simulink model "MR11Simulinknodos"  (R2013a)
settings: Solver=ode45  StartTime=0.0  StopTime=10.0  RelTol=1e-3
libraries: powerlib x63
settings Model: Creator=Erika  LastModifiedBy=Erika

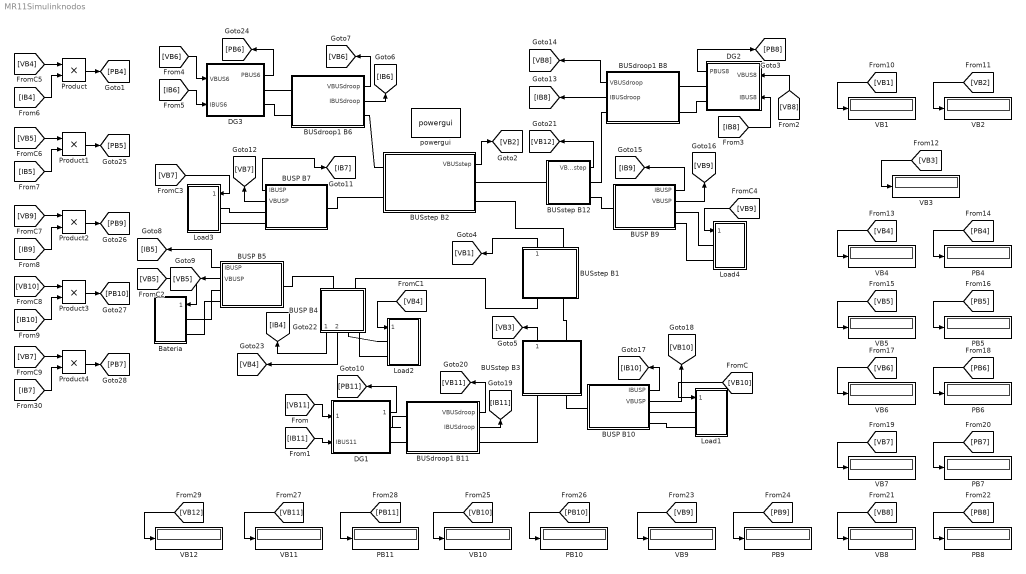
== system MR11Simulinknodos ==
  BUSP B10 : Subsystem
  BUSP B4 : Subsystem
  BUSP B5 : Subsystem
  BUSP B7 : Subsystem
  BUSP B9 : Subsystem
  BUSdroop1 B11 : Subsystem
  BUSdroop1 B6 : Subsystem
  BUSdroop1 B8 : Subsystem
  BUSstep B1 : Subsystem
  BUSstep B12 : Subsystem
  BUSstep B2 : Subsystem
  BUSstep B3 : Subsystem
  Bateria : Subsystem
  DG1 : Subsystem
  DG2 : Subsystem
  DG3 : Subsystem
  Load1 : Subsystem
  Load2 : Subsystem
  Load3 : Subsystem
  Load4 : Subsystem
  PB{4..11} (8 alike) : Display
  Product{,1..4} (5 alike) : Product
  VB{1..12} (12 alike) : Display
  powergui : powerlib/powergui  Priority=1  SimulationMode=Continuous  SolverType=Tustin  SampleTime=50e-6  frequency=60  SPID=off  DisableSnubberDevices=off  DisableRonSwitches=off  DisableVfSwitches=off  SwTol=0  Interpol=off  DisplayEquations=off  frequencyindice=0  Pbase=100e6  ErrMax=1e-4  Iterations=50  UnitsV=kV  UnitsW=MW  FunctionMessages=off  echomessages=off  HookPort=off  EnableUseOfTLC=off  x0status=blocks  RestoreLinks=warning  ResistiveCurrentMeasurement=off  Frange=[0:2:500]  Ylog=off  Xlog=on  ShowGrid=off  save=off  variable=ZData  ZoomFFT=off  StartTime=0.0  cycles=1  DisplayStyle=1  fundamental=60  FreqAxis=off  MaxFrequency=1000  frequencyindicesteady=1  RmsSteady=1  display=off  Ts=0  methode=off
  wires:
  [VB11] -> DG1/1(VBUS11)
  [IB11] -> DG1/2(IBUS11)
  DG1/1(PBUS11) -> [PB11]
  BUSP B5/1(IBUSP) -> [IB5]
  BUSP B5/2(VBUSP) -> [VB5]
  [VB10] -> Load1/1(VBUSc)
  BUSstep B1/1(VBUSstep) -> [VB1]
  BUSstep B2/1(VBUSstep) -> [VB2]
  BUSstep B3/1(VBUSstep) -> [VB3]
  BUSdroop1 B6/1(VBUSdroop) -> [VB6]
  BUSdroop1 B6/2(IBUSdroop) -> [IB6]
  BUSP B7/1(IBUSP) -> [IB7]
  BUSP B7/2(VBUSP) -> [VB7]
  BUSdroop1 B8/1(VBUSdroop) -> [VB8]
  BUSdroop1 B8/2(IBUSdroop) -> [IB8]
  BUSP B9/1(IBUSP) -> [IB9]
  BUSP B9/2(VBUSP) -> [VB9]
  BUSP B10/1(IBUSP) -> [IB10]
  BUSP B10/2(VBUSP) -> [VB10]
  BUSdroop1 B11/1(VBUSdroop) -> [VB11]
  BUSdroop1 B11/2(IBUSdroop) -> [IB11]
  BUSstep B12/1(VBUSstep) -> [VB12]
  BUSP B4/1(IBUSP) -> [IB4]
  BUSP B4/2(VBUSP) -> [VB4]
  [VB8] -> DG2/1(VBUS8)
  [IB8] -> DG2/2(IBUS8)
  DG2/1(PBUS8) -> [PB8]
  [VB6] -> DG3/1(VBUS6)
  [IB6] -> DG3/2(IBUS6)
  DG3/1(PBUS6) -> [PB6]
  [VB4] -> Load2/1(VBUSc)
  [VB5] -> Bateria/1(VBUSc)
  [VB7] -> Load3/1(VBUSc)
  [VB9] -> Load4/1(VBUSc)
  [VB4] -> Product/1
  [IB4] -> Product/2
  Product/1 -> [PB4]
  [VB5] -> Product1/1
  [IB5] -> Product1/2
  Product1/1 -> [PB5]
  [VB9] -> Product2/1
  [IB9] -> Product2/2
  Product2/1 -> [PB9]
  [VB10] -> Product3/1
  [IB10] -> Product3/2
  Product3/1 -> [PB10]
  [VB1] -> VB1/1
  [VB2] -> VB2/1
  [VB3] -> VB3/1
  [VB4] -> VB4/1
  [PB4] -> PB4/1
  [VB5] -> VB5/1
  [PB5] -> PB5/1
  [VB6] -> VB6/1
  [PB6] -> PB6/1
  [VB7] -> VB7/1
  [PB7] -> PB7/1
  [VB8] -> VB8/1
  [PB8] -> PB8/1
  [VB9] -> VB9/1
  [PB9] -> PB9/1
  [VB10] -> VB10/1
  [PB10] -> PB10/1
  [VB11] -> VB11/1
  [PB11] -> PB11/1
  [VB12] -> VB12/1
  [VB7] -> Product4/1
  [IB7] -> Product4/2
  Product4/1 -> [PB7]
  connections:
  BUSstep B1/RConn1 -- BUSstep B2/RConn2
  BUSstep B1/LConn1 -- BUSP B4/LConn2
  BUSstep B1/LConn2 -- BUSstep B3/RConn1
  BUSstep B2/RConn1 -- BUSstep B12/LConn1
  BUSstep B12/RConn2 -- BUSP B9/LConn1
  BUSstep B12/RConn1 -- BUSdroop1 B8/RConn1
  BUSstep B2/LConn1 -- BUSdroop1 B6/RConn1
  BUSstep B2/LConn2 -- BUSP B7/LConn1
  BUSP B4/LConn1 -- BUSP B5/LConn1
  BUSstep B3/LConn1 -- BUSdroop1 B11/RConn1
  BUSstep B3/LConn2 -- BUSP B10/LConn1
  DG1/RConn1 -- BUSdroop1 B11/LConn1
  DG1/RConn2 -- BUSdroop1 B11/LConn2
  DG2/RConn1 -- BUSdroop1 B8/LConn1
  DG2/RConn2 -- BUSdroop1 B8/LConn2
  DG3/RConn1 -- BUSdroop1 B6/LConn1
  DG3/RConn2 -- BUSdroop1 B6/LConn2
  Load1/LConn1 -- BUSP B10/RConn1
  Load1/LConn2 -- BUSP B10/RConn2
  Load2/LConn2 -- BUSP B4/RConn2
  Load2/LConn1 -- BUSP B4/RConn1
  Bateria/LConn1 -- BUSP B5/RConn1
  Bateria/LConn2 -- BUSP B5/RConn2
  Load3/LConn2 -- BUSP B7/RConn2
  Load3/LConn1 -- BUSP B7/RConn1
  Load4/LConn1 -- BUSP B9/RConn1
  Load4/LConn2 -- BUSP B9/RConn2

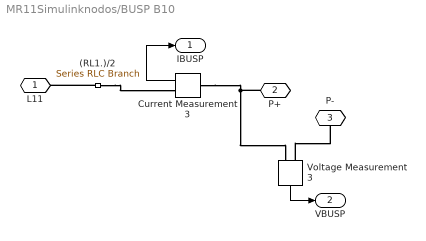
== system MR11Simulinknodos/BUSP B10 ==
  (RL1.)/2 : powerlib/Elements/Series RLC Branch  LConnTagsString=__new0  RConnTagsString=__new0  BranchType=R  Resistance=0.09  Inductance=1e-3  SetiL0=off  InitialCurrent=0  Capacitance=1e-6  Setx0=off  InitialVoltage=0  Measurements=None
  Current Measurement3 : powerlib/Measurements/Current Measurement  PhasorSimulation=off  OutputType=Complex  PSBequivalent=0
  Voltage Measurement3 : powerlib/Measurements/Voltage Measurement  PhasorSimulation=off  OutputType=Complex  PSBequivalent=0
  L11 : PMIOPort  Port=1  Side=Left
  P+ : PMIOPort  Port=2  Side=Right
  P- : PMIOPort  Port=3  Side=Right
  IBUSP : Outport
  VBUSP : Outport  Port=2
  wires:
  Current Measurement3/1 -> IBUSP/1
  Voltage Measurement3/1 -> VBUSP/1
  connections:
  Voltage Measurement3/LConn2 -- P-/RConn1
  (RL1.)/2/LConn1 -- L11/RConn1
  (RL1.)/2/RConn1 -- Current Measurement3/RConn1
  Current Measurement3/LConn1 -- Voltage Measurement3/LConn1 -- P+/RConn1

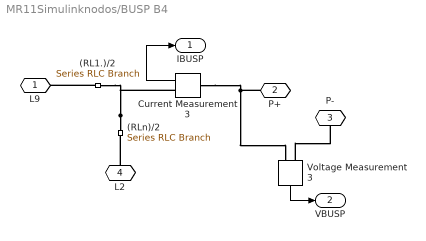
== system MR11Simulinknodos/BUSP B4 ==
  (RL1.)/2 : powerlib/Elements/Series RLC Branch  LConnTagsString=__new0  RConnTagsString=__new0  BranchType=R  Resistance=0.1  Inductance=1e-3  SetiL0=off  InitialCurrent=0  Capacitance=1e-6  Setx0=off  InitialVoltage=0  Measurements=None
  (RLn)/2 : powerlib/Elements/Series RLC Branch  LConnTagsString=__new0  RConnTagsString=__new0  BranchType=R  Resistance=0.2  Inductance=1e-3  SetiL0=off  InitialCurrent=0  Capacitance=1e-6  Setx0=off  InitialVoltage=0  Measurements=None
  Current Measurement3 : powerlib/Measurements/Current Measurement  PhasorSimulation=off  OutputType=Complex  PSBequivalent=0
  Voltage Measurement3 : powerlib/Measurements/Voltage Measurement  PhasorSimulation=off  OutputType=Complex  PSBequivalent=0
  L9 : PMIOPort  Port=1  Side=Left
  P+ : PMIOPort  Port=2  Side=Right
  P- : PMIOPort  Port=3  Side=Right
  L2 : PMIOPort  Port=4  Side=Left
  IBUSP : Outport
  VBUSP : Outport  Port=2
  wires:
  Current Measurement3/1 -> IBUSP/1
  Voltage Measurement3/1 -> VBUSP/1
  connections:
  Voltage Measurement3/LConn2 -- P-/RConn1
  L2/RConn1 -- (RLn)/2/RConn1
  (RL1.)/2/LConn1 -- L9/RConn1
  (RLn)/2/LConn1 -- Current Measurement3/RConn1 -- (RL1.)/2/RConn1
  Current Measurement3/LConn1 -- Voltage Measurement3/LConn1 -- P+/RConn1

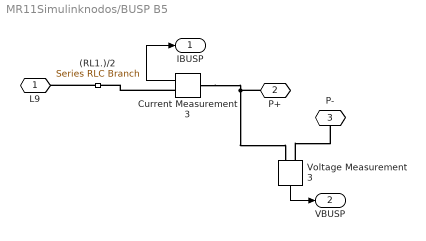
== system MR11Simulinknodos/BUSP B5 ==
  (RL1.)/2 : powerlib/Elements/Series RLC Branch  LConnTagsString=__new0  RConnTagsString=__new0  BranchType=R  Resistance=0.1  Inductance=1e-3  SetiL0=off  InitialCurrent=0  Capacitance=1e-6  Setx0=off  InitialVoltage=0  Measurements=None
  Current Measurement3 : powerlib/Measurements/Current Measurement  PhasorSimulation=off  OutputType=Complex  PSBequivalent=0
  Voltage Measurement3 : powerlib/Measurements/Voltage Measurement  PhasorSimulation=off  OutputType=Complex  PSBequivalent=0
  L9 : PMIOPort  Port=1  Side=Left
  P+ : PMIOPort  Port=2  Side=Right
  P- : PMIOPort  Port=3  Side=Right
  IBUSP : Outport
  VBUSP : Outport  Port=2
  wires:
  Voltage Measurement3/1 -> VBUSP/1
  Current Measurement3/1 -> IBUSP/1
  connections:
  P+/RConn1 -- Voltage Measurement3/LConn1 -- Current Measurement3/LConn1
  Current Measurement3/RConn1 -- (RL1.)/2/RConn1
  (RL1.)/2/LConn1 -- L9/RConn1
  Voltage Measurement3/LConn2 -- P-/RConn1

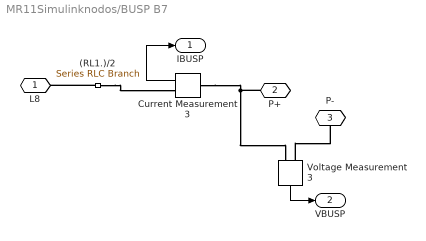
== system MR11Simulinknodos/BUSP B7 ==
  (RL1.)/2 : powerlib/Elements/Series RLC Branch  LConnTagsString=__new0  RConnTagsString=__new0  BranchType=R  Resistance=0.07  Inductance=1e-3  SetiL0=off  InitialCurrent=0  Capacitance=1e-6  Setx0=off  InitialVoltage=0  Measurements=None
  Current Measurement3 : powerlib/Measurements/Current Measurement  PhasorSimulation=off  OutputType=Complex  PSBequivalent=0
  Voltage Measurement3 : powerlib/Measurements/Voltage Measurement  PhasorSimulation=off  OutputType=Complex  PSBequivalent=0
  L8 : PMIOPort  Port=1  Side=Left
  P+ : PMIOPort  Port=2  Side=Right
  P- : PMIOPort  Port=3  Side=Right
  IBUSP : Outport
  VBUSP : Outport  Port=2
  wires:
  Current Measurement3/1 -> IBUSP/1
  Voltage Measurement3/1 -> VBUSP/1
  connections:
  Voltage Measurement3/LConn2 -- P-/RConn1
  (RL1.)/2/LConn1 -- L8/RConn1
  (RL1.)/2/RConn1 -- Current Measurement3/RConn1
  Current Measurement3/LConn1 -- Voltage Measurement3/LConn1 -- P+/RConn1

== system MR11Simulinknodos/BUSP B9 ==
  (RLn)/2 : powerlib/Elements/Series RLC Branch  LConnTagsString=__new0  RConnTagsString=__new0  BranchType=R  Resistance=0.05  Inductance=1e-3  SetiL0=off  InitialCurrent=0  Capacitance=1e-6  Setx0=off  InitialVoltage=0  Measurements=None
  Current Measurement3 : powerlib/Measurements/Current Measurement  PhasorSimulation=off  OutputType=Complex  PSBequivalent=0
  Voltage Measurement3 : powerlib/Measurements/Voltage Measurement  PhasorSimulation=off  OutputType=Complex  PSBequivalent=0
  P+ : PMIOPort  Port=1  Side=Right
  P- : PMIOPort  Port=2  Side=Right
  L5 : PMIOPort  Port=3  Side=Left
  IBUSP : Outport
  VBUSP : Outport  Port=2
  wires:
  Voltage Measurement3/1 -> VBUSP/1
  Current Measurement3/1 -> IBUSP/1
  connections:
  P+/RConn1 -- Voltage Measurement3/LConn1 -- Current Measurement3/LConn1
  Current Measurement3/RConn1 -- (RLn)/2/LConn1
  L5/RConn1 -- (RLn)/2/RConn1
  Voltage Measurement3/LConn2 -- P-/RConn1

== system MR11Simulinknodos/BUSdroop1 B11 ==
  " (RL1)/2" : powerlib/Elements/Series RLC Branch  LConnTagsString=__new0  RConnTagsString=__new0  BranchType=R  Resistance=0.15  Inductance=1e-3  SetiL0=off  InitialCurrent=0  Capacitance=1e-6  Setx0=off  InitialVoltage=0  Measurements=None
  Current Measurement : powerlib/Measurements/Current Measurement  PhasorSimulation=off  OutputType=Complex  PSBequivalent=0
  Voltage Measurement : powerlib/Measurements/Voltage Measurement  PhasorSimulation=off  OutputType=Complex  PSBequivalent=0
  L10 : PMIOPort  Port=1  Side=Right
  DG1+ : PMIOPort  Port=2  Side=Left
  DG1- : PMIOPort  Port=3  Side=Left
  VBUSdroop : Outport
  IBUSdroop : Outport  Port=2
  wires:
  Voltage Measurement/1 -> VBUSdroop/1
  Current Measurement/1 -> IBUSdroop/1
  connections:
  " (RL1)/2"/RConn1 -- L10/RConn1
  Current Measurement/LConn1 -- DG1+/RConn1 -- Voltage Measurement/LConn1
  " (RL1)/2"/LConn1 -- Current Measurement/RConn1
  Voltage Measurement/LConn2 -- DG1-/RConn1

== system MR11Simulinknodos/BUSdroop1 B6 ==
  " (RL1)/2" : powerlib/Elements/Series RLC Branch  LConnTagsString=__new0  RConnTagsString=__new0  BranchType=R  Resistance=0.08  Inductance=1e-3  SetiL0=off  InitialCurrent=0  Capacitance=1e-6  Setx0=off  InitialVoltage=0  Measurements=None
  Current Measurement : powerlib/Measurements/Current Measurement  PhasorSimulation=off  OutputType=Complex  PSBequivalent=0
  Voltage Measurement : powerlib/Measurements/Voltage Measurement  PhasorSimulation=off  OutputType=Complex  PSBequivalent=0
  L7 : PMIOPort  Port=1  Side=Right
  DG3+ : PMIOPort  Port=2  Side=Left
  DG3- : PMIOPort  Port=3  Side=Left
  VBUSdroop : Outport
  IBUSdroop : Outport  Port=2
  wires:
  Current Measurement/1 -> IBUSdroop/1
  Voltage Measurement/1 -> VBUSdroop/1
  connections:
  Voltage Measurement/LConn2 -- DG3-/RConn1
  " (RL1)/2"/LConn1 -- Current Measurement/RConn1
  Voltage Measurement/LConn1 -- DG3+/RConn1 -- Current Measurement/LConn1
  " (RL1)/2"/RConn1 -- L7/RConn1

== system MR11Simulinknodos/BUSdroop1 B8 ==
  " (RL1)/2" : powerlib/Elements/Series RLC Branch  LConnTagsString=__new0  RConnTagsString=__new0  BranchType=R  Resistance=0.2  Inductance=1e-3  SetiL0=off  InitialCurrent=0  Capacitance=1e-6  Setx0=off  InitialVoltage=0  Measurements=None
  Current Measurement : powerlib/Measurements/Current Measurement  PhasorSimulation=off  OutputType=Complex  PSBequivalent=0
  Voltage Measurement : powerlib/Measurements/Voltage Measurement  PhasorSimulation=off  OutputType=Complex  PSBequivalent=0
  L6 : PMIOPort  Port=1  Side=Right
  DG2+ : PMIOPort  Port=2  Side=Left
  DG2- : PMIOPort  Port=3  Side=Left
  VBUSdroop : Outport
  IBUSdroop : Outport  Port=2
  wires:
  Voltage Measurement/1 -> VBUSdroop/1
  Current Measurement/1 -> IBUSdroop/1
  connections:
  " (RL1)/2"/RConn1 -- L6/RConn1
  Current Measurement/LConn1 -- DG2+/RConn1 -- Voltage Measurement/LConn1
  " (RL1)/2"/LConn1 -- Current Measurement/RConn1
  Voltage Measurement/LConn2 -- DG2-/RConn1

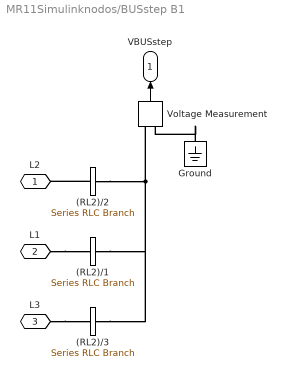
== system MR11Simulinknodos/BUSstep B1 ==
  " (RL2)/1" : powerlib/Elements/Series RLC Branch  LConnTagsString=__new0  RConnTagsString=__new0  BranchType=R  Resistance=0.35  Inductance=1e-3  SetiL0=off  InitialCurrent=0  Capacitance=1e-6  Setx0=off  InitialVoltage=0  Measurements=None
  " (RL2)/2" : powerlib/Elements/Series RLC Branch  LConnTagsString=__new0  RConnTagsString=__new0  BranchType=R  Resistance=0.2  Inductance=1e-3  SetiL0=off  InitialCurrent=0  Capacitance=1e-6  Setx0=off  InitialVoltage=0  Measurements=None
  " (RL2)/3" : powerlib/Elements/Series RLC Branch  LConnTagsString=__new0  RConnTagsString=__new0  BranchType=R  Resistance=0.3  Inductance=1e-3  SetiL0=off  InitialCurrent=0  Capacitance=1e-6  Setx0=off  InitialVoltage=0  Measurements=None
  Ground : powerlib/Elements/Ground  LConnTagsString=a
  Voltage Measurement : powerlib/Measurements/Voltage Measurement  PhasorSimulation=off  OutputType=Complex  PSBequivalent=0
  L2 : PMIOPort  Port=1  Side=Left
  L1 : PMIOPort  Port=2  Side=Left
  L3 : PMIOPort  Port=3  Side=Right
  VBUSstep : Outport
  wires:
  Voltage Measurement/1 -> VBUSstep/1
  connections:
  " (RL2)/2"/LConn1 -- L2/RConn1
  Ground/LConn1 -- Voltage Measurement/LConn2
  " (RL2)/2"/RConn1 -- " (RL2)/3"/RConn1 -- " (RL2)/1"/RConn1 -- Voltage Measurement/LConn1
  L1/RConn1 -- " (RL2)/1"/LConn1
  L3/RConn1 -- " (RL2)/3"/LConn1

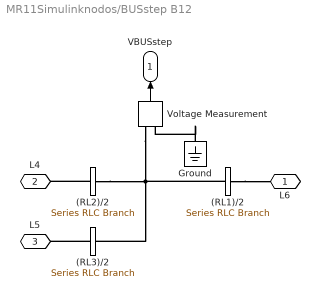
== system MR11Simulinknodos/BUSstep B12 ==
  " (RL1)/2" : powerlib/Elements/Series RLC Branch  LConnTagsString=__new0  RConnTagsString=__new0  BranchType=R  Resistance=0.2  Inductance=1e-3  SetiL0=off  InitialCurrent=0  Capacitance=1e-6  Setx0=off  InitialVoltage=0  Measurements=None
  " (RL2)/2" : powerlib/Elements/Series RLC Branch  LConnTagsString=__new0  RConnTagsString=__new0  BranchType=R  Resistance=0.1  Inductance=1e-3  SetiL0=off  InitialCurrent=0  Capacitance=1e-6  Setx0=off  InitialVoltage=0  Measurements=None
  " (RL3)/2" : powerlib/Elements/Series RLC Branch  LConnTagsString=__new0  RConnTagsString=__new0  BranchType=R  Resistance=0.05  Inductance=1e-3  SetiL0=off  InitialCurrent=0  Capacitance=1e-6  Setx0=off  InitialVoltage=0  Measurements=None
  Ground : powerlib/Elements/Ground  LConnTagsString=a
  Voltage Measurement : powerlib/Measurements/Voltage Measurement  PhasorSimulation=off  OutputType=Complex  PSBequivalent=0
  L6 : PMIOPort  Port=1  Side=Right
  L4 : PMIOPort  Port=2  Side=Left
  L5 : PMIOPort  Port=3  Side=Right
  VBUSstep : Outport
  wires:
  Voltage Measurement/1 -> VBUSstep/1
  connections:
  " (RL1)/2"/RConn1 -- L6/RConn1
  " (RL3)/2"/LConn1 -- L5/RConn1
  " (RL2)/2"/LConn1 -- L4/RConn1
  Ground/LConn1 -- Voltage Measurement/LConn2
  Voltage Measurement/LConn1 -- " (RL2)/2"/RConn1 -- " (RL1)/2"/LConn1 -- " (RL3)/2"/RConn1

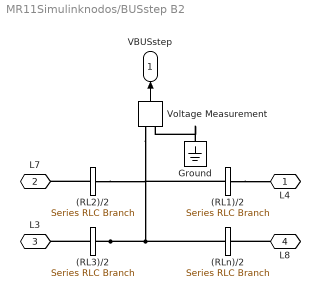
== system MR11Simulinknodos/BUSstep B2 ==
  " (RL1)/2" : powerlib/Elements/Series RLC Branch  LConnTagsString=__new0  RConnTagsString=__new0  BranchType=R  Resistance=0.1  Inductance=1e-3  SetiL0=off  InitialCurrent=0  Capacitance=1e-6  Setx0=off  InitialVoltage=0  Measurements=None
  " (RL2)/2" : powerlib/Elements/Series RLC Branch  LConnTagsString=__new0  RConnTagsString=__new0  BranchType=R  Resistance=0.08  Inductance=1e-3  SetiL0=off  InitialCurrent=0  Capacitance=1e-6  Setx0=off  InitialVoltage=0  Measurements=None
  " (RL3)/2" : powerlib/Elements/Series RLC Branch  LConnTagsString=__new0  RConnTagsString=__new0  BranchType=R  Resistance=0.3  Inductance=1e-3  SetiL0=off  InitialCurrent=0  Capacitance=1e-6  Setx0=off  InitialVoltage=0  Measurements=None
  " (RLn)/2" : powerlib/Elements/Series RLC Branch  LConnTagsString=__new0  RConnTagsString=__new0  BranchType=R  Resistance=0.07  Inductance=1e-3  SetiL0=off  InitialCurrent=0  Capacitance=1e-6  Setx0=off  InitialVoltage=0  Measurements=None
  Ground : powerlib/Elements/Ground  LConnTagsString=a
  Voltage Measurement : powerlib/Measurements/Voltage Measurement  PhasorSimulation=off  OutputType=Complex  PSBequivalent=0
  L4 : PMIOPort  Port=1  Side=Right
  L7 : PMIOPort  Port=2  Side=Left
  L3 : PMIOPort  Port=3  Side=Right
  L8 : PMIOPort  Port=4  Side=Left
  VBUSstep : Outport
  wires:
  Voltage Measurement/1 -> VBUSstep/1
  connections:
  L8/RConn1 -- " (RLn)/2"/RConn1
  " (RL3)/2"/RConn1 -- " (RLn)/2"/LConn1 -- " (RL1)/2"/LConn1 -- " (RL2)/2"/RConn1 -- Voltage Measurement/LConn1
  Ground/LConn1 -- Voltage Measurement/LConn2
  " (RL2)/2"/LConn1 -- L7/RConn1
  " (RL3)/2"/LConn1 -- L3/RConn1
  " (RL1)/2"/RConn1 -- L4/RConn1

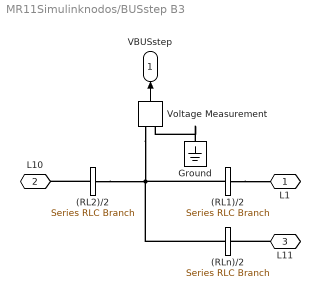
== system MR11Simulinknodos/BUSstep B3 ==
  " (RL1)/2" : powerlib/Elements/Series RLC Branch  LConnTagsString=__new0  RConnTagsString=__new0  BranchType=R  Resistance=0.35  Inductance=1e-3  SetiL0=off  InitialCurrent=0  Capacitance=1e-6  Setx0=off  InitialVoltage=0  Measurements=None
  " (RL2)/2" : powerlib/Elements/Series RLC Branch  LConnTagsString=__new0  RConnTagsString=__new0  BranchType=R  Resistance=0.15  Inductance=1e-3  SetiL0=off  InitialCurrent=0  Capacitance=1e-6  Setx0=off  InitialVoltage=0  Measurements=None
  " (RLn)/2" : powerlib/Elements/Series RLC Branch  LConnTagsString=__new0  RConnTagsString=__new0  BranchType=R  Resistance=0.09  Inductance=1e-3  SetiL0=off  InitialCurrent=0  Capacitance=1e-6  Setx0=off  InitialVoltage=0  Measurements=None
  Ground : powerlib/Elements/Ground  LConnTagsString=a
  Voltage Measurement : powerlib/Measurements/Voltage Measurement  PhasorSimulation=off  OutputType=Complex  PSBequivalent=0
  L1 : PMIOPort  Port=1  Side=Right
  L10 : PMIOPort  Port=2  Side=Left
  L11 : PMIOPort  Port=3  Side=Left
  VBUSstep : Outport
  wires:
  Voltage Measurement/1 -> VBUSstep/1
  connections:
  " (RL1)/2"/RConn1 -- L1/RConn1
  " (RL2)/2"/LConn1 -- L10/RConn1
  Ground/LConn1 -- Voltage Measurement/LConn2
  Voltage Measurement/LConn1 -- " (RLn)/2"/LConn1 -- " (RL2)/2"/RConn1 -- " (RL1)/2"/LConn1
  L11/RConn1 -- " (RLn)/2"/RConn1

== system MR11Simulinknodos/Bateria ==
  VBUSc : Inport
  Constant4 : Constant  Value=-10000
  Controlled Current Source : powerlib/Electrical Sources/Controlled Current Source  Initialize=off  Source_Type=DC  Amplitude=0  Phase=0  Frequency=0  Measurements=None
  Divide2 : Product  Inputs=*/
  Ground3 : powerlib/Elements/Ground  LConnTagsString=a
  Bat+ : PMIOPort  Port=1  Side=Left
  Bat1- : PMIOPort  Port=2  Side=Left
  wires:
  Constant4/1 -> Divide2/1
  Divide2/1 -> Controlled Current Source/1
  VBUSc/1 -> Divide2/2
  connections:
  Controlled Current Source/RConn1 -- Bat1-/RConn1 -- Ground3/LConn1
  Controlled Current Source/LConn1 -- Bat+/RConn1

== system MR11Simulinknodos/DG1 ==
  VBUS11 : Inport
  IBUS11 : Inport  Port=2
  DroopDG1 : Subsystem
  G1 : powerlib/Electrical Sources/Controlled Voltage Source  Initialize=on  Source_Type=DC  Amplitude=500  Phase=0  Frequency=0  Measurements=None
  Ground : powerlib/Elements/Ground  LConnTagsString=a
  DG1+ : PMIOPort  Port=1  Side=Right
  DG1- : PMIOPort  Port=2  Side=Right
  PBUS11 : Outport
  wires:
  DroopDG1/1(Vdroop1) -> G1/1
  DroopDG1/2(PDG1) -> PBUS11/1
  IBUS11/1 -> DroopDG1/2(IG1)
  VBUS11/1 -> DroopDG1/1(VG1)
  connections:
  G1/LConn1 -- DG1-/RConn1 -- Ground/LConn1
  DG1+/RConn1 -- G1/RConn1

== system MR11Simulinknodos/DG2 ==
  VBUS8 : Inport
  IBUS8 : Inport  Port=2
  DroopDG1 : Subsystem
  G1 : powerlib/Electrical Sources/Controlled Voltage Source  Initialize=on  Source_Type=DC  Amplitude=500  Phase=0  Frequency=0  Measurements=None
  Ground : powerlib/Elements/Ground  LConnTagsString=a
  DG2+ : PMIOPort  Port=1  Side=Right
  DG2- : PMIOPort  Port=2  Side=Right
  PBUS8 : Outport
  wires:
  VBUS8/1 -> DroopDG1/1(VG1)
  IBUS8/1 -> DroopDG1/2(IG1)
  DroopDG1/2(PDG1) -> PBUS8/1
  DroopDG1/1(Vdroop1) -> G1/1
  connections:
  DG2+/RConn1 -- G1/RConn1
  Ground/LConn1 -- DG2-/RConn1 -- G1/LConn1

== system MR11Simulinknodos/DG3 ==
  VBUS6 : Inport
  IBUS6 : Inport  Port=2
  DroopDG1 : Subsystem
  G1 : powerlib/Electrical Sources/Controlled Voltage Source  Initialize=on  Source_Type=DC  Amplitude=500  Phase=0  Frequency=0  Measurements=None
  Ground : powerlib/Elements/Ground  LConnTagsString=a
  DG3+ : PMIOPort  Port=1  Side=Right
  DG3- : PMIOPort  Port=2  Side=Right
  PBUS6 : Outport
  wires:
  VBUS6/1 -> DroopDG1/1(VG1)
  IBUS6/1 -> DroopDG1/2(IG1)
  DroopDG1/2(PDG1) -> PBUS6/1
  DroopDG1/1(Vdroop1) -> G1/1
  connections:
  DG3+/RConn1 -- G1/RConn1
  Ground/LConn1 -- DG3-/RConn1 -- G1/LConn1

== system MR11Simulinknodos/Load1 ==
  VBUSc : Inport
  Constant4 : Constant  Value=20800
  Controlled Current Source : powerlib/Electrical Sources/Controlled Current Source  Initialize=off  Source_Type=DC  Amplitude=0  Phase=0  Frequency=0  Measurements=None
  Divide2 : Product  Inputs=*/
  Ground3 : powerlib/Elements/Ground  LConnTagsString=a
  Load1+ : PMIOPort  Port=1  Side=Left
  Load1- : PMIOPort  Port=2  Side=Left
  wires:
  Constant4/1 -> Divide2/1
  Divide2/1 -> Controlled Current Source/1
  VBUSc/1 -> Divide2/2
  connections:
  Controlled Current Source/RConn1 -- Load1-/RConn1 -- Ground3/LConn1
  Controlled Current Source/LConn1 -- Load1+/RConn1

== system MR11Simulinknodos/Load2 ==
  VBUSc : Inport
  Constant4 : Constant  Value=11300
  Controlled Current Source : powerlib/Electrical Sources/Controlled Current Source  Initialize=off  Source_Type=DC  Amplitude=0  Phase=0  Frequency=0  Measurements=None
  Divide2 : Product  Inputs=*/
  Ground3 : powerlib/Elements/Ground  LConnTagsString=a
  Load1+ : PMIOPort  Port=1  Side=Left
  Load1- : PMIOPort  Port=2  Side=Left
  wires:
  VBUSc/1 -> Divide2/2
  Divide2/1 -> Controlled Current Source/1
  Constant4/1 -> Divide2/1
  connections:
  Controlled Current Source/LConn1 -- Load1+/RConn1
  Ground3/LConn1 -- Load1-/RConn1 -- Controlled Current Source/RConn1

== system MR11Simulinknodos/Load3 ==
  VBUSc : Inport
  Constant4 : Constant  Value=16700
  Controlled Current Source : powerlib/Electrical Sources/Controlled Current Source  Initialize=off  Source_Type=DC  Amplitude=0  Phase=0  Frequency=0  Measurements=None
  Divide2 : Product  Inputs=*/
  Ground3 : powerlib/Elements/Ground  LConnTagsString=a
  Load1+ : PMIOPort  Port=1  Side=Left
  Load1- : PMIOPort  Port=2  Side=Left
  wires:
  Constant4/1 -> Divide2/1
  Divide2/1 -> Controlled Current Source/1
  VBUSc/1 -> Divide2/2
  connections:
  Controlled Current Source/RConn1 -- Load1-/RConn1 -- Ground3/LConn1
  Controlled Current Source/LConn1 -- Load1+/RConn1

== system MR11Simulinknodos/Load4 ==
  VBUSc : Inport
  Constant4 : Constant  Value=20800
  Controlled Current Source : powerlib/Electrical Sources/Controlled Current Source  Initialize=off  Source_Type=DC  Amplitude=0  Phase=0  Frequency=0  Measurements=None
  Divide2 : Product  Inputs=*/
  Ground3 : powerlib/Elements/Ground  LConnTagsString=a
  Load1+ : PMIOPort  Port=1  Side=Left
  Load1- : PMIOPort  Port=2  Side=Left
  wires:
  Constant4/1 -> Divide2/1
  Divide2/1 -> Controlled Current Source/1
  VBUSc/1 -> Divide2/2
  connections:
  Controlled Current Source/RConn1 -- Load1-/RConn1 -- Ground3/LConn1
  Controlled Current Source/LConn1 -- Load1+/RConn1

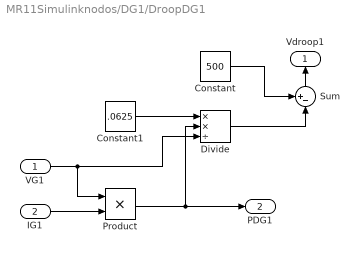
== system MR11Simulinknodos/DG1/DroopDG1 ==
  VG1 : Inport
  IG1 : Inport  Port=2
  Constant : Constant  Value=500
  Constant1 : Constant  Value=.0625
  Divide : Product  Inputs=**/
  Product : Product
  Sum : Sum  Inputs=+-|
  Vdroop1 : Outport
  PDG1 : Outport  Port=2
  wires:
  Constant1/1 -> Divide/1
  IG1/1 -> Product/2
  Constant/1 -> Sum/1
  Sum/1 -> Vdroop1/1
  Divide/1 -> Sum/2
  VG1/1 -> Product/1, Divide/3
  Product/1 -> Divide/2, PDG1/1

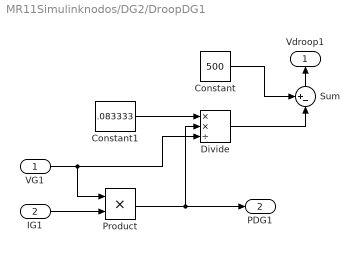
== system MR11Simulinknodos/DG2/DroopDG1 ==
  VG1 : Inport
  IG1 : Inport  Port=2
  Constant : Constant  Value=500
  Constant1 : Constant  Value=.083333
  Divide : Product  Inputs=**/
  Product : Product
  Sum : Sum  Inputs=+-|
  Vdroop1 : Outport
  PDG1 : Outport  Port=2
  wires:
  Product/1 -> PDG1/1, Divide/2
  VG1/1 -> Divide/3, Product/1
  Divide/1 -> Sum/2
  Sum/1 -> Vdroop1/1
  Constant/1 -> Sum/1
  IG1/1 -> Product/2
  Constant1/1 -> Divide/1

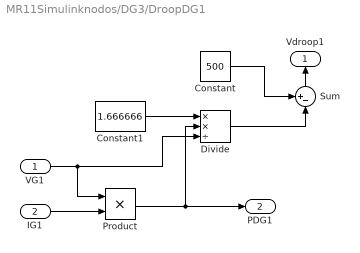
== system MR11Simulinknodos/DG3/DroopDG1 ==
  VG1 : Inport
  IG1 : Inport  Port=2
  Constant : Constant  Value=500
  Constant1 : Constant  Value=1.666666
  Divide : Product  Inputs=**/
  Product : Product
  Sum : Sum  Inputs=+-|
  Vdroop1 : Outport
  PDG1 : Outport  Port=2
  wires:
  Product/1 -> PDG1/1, Divide/2
  VG1/1 -> Divide/3, Product/1
  Divide/1 -> Sum/2
  Sum/1 -> Vdroop1/1
  Constant/1 -> Sum/1
  IG1/1 -> Product/2
  Constant1/1 -> Divide/1
